simulink model "GammaandTorqueMover"  (R2022b)
settings: Solver=FixedStepAuto  StartTime=0.0  StopTime=10  FixedStep=0.01  RelTol=1e-3
undefined symbols (not defined in the file or in its folder): Kd, Ki, Kp
libraries: mpclib x6, slpidlib x6, simulink x1
(part 3 of 4)

== matlab function GammaandTorqueMover/PID/Subsystem/PINV/GAMMA ==
  data: input input; position input; output output; TAU input; BETA_K input; ALPHA_X input; ALPHA_Y input; ALPHA_Z input; ALPHA_M1 input; ALPHA_M2 input; BETA_M1 input; BETA_M2 input; ALPHA_RZ input; PI input
function output = computeGammaPinvBlock(input,position,TAU,BETA_K,ALPHA_X,ALPHA_Y,ALPHA_Z,ALPHA_M1,ALPHA_M2,BETA_M1,BETA_M2,ALPHA_RZ,PI)
    % Call the generated function to compute Gamma
    X_M = position(1);
    Y_M = position(2);
    Z_M = position(3);
    ALPHA_ROTATION_M = position(4);
    BETA_ROTATION_M = position(5);
    GAMMA_ROTATION_M = position(6);
    Gamma = computeFullGammawithTorqueR4(X_M,Y_M,Z_M,ALPHA_ROTATION_M,BETA_ROTATION_M,GAMMA_ROTATION_M,TAU,BETA_K,ALPHA_X,ALPHA_Y,ALPHA_Z,ALPHA_M1,ALPHA_M2,BETA_M1,BETA_M2,ALPHA_RZ,PI);
    Gamma_pinv = pinv(Gamma);
    
    % Multiply Gamma by the input
    output =Gamma_pinv * input ;
end

== matlab function GammaandTorqueMover/Open loop system/Subsystem/Gamma/GAMMA ==
  data: input input; position input; output output; TAU input; BETA_K input; ALPHA_X input; ALPHA_Y input; ALPHA_Z input; ALPHA_M1 input; ALPHA_M2 input; BETA_M1 input; BETA_M2 input; ALPHA_RZ input; PI input
function output = computeGammaBlock(input, position,TAU,BETA_K,ALPHA_X,ALPHA_Y,ALPHA_Z,ALPHA_M1,ALPHA_M2,BETA_M1,BETA_M2,ALPHA_RZ,PI)
% Call the generated function to compute Gamma
    X_M = position(1);
    Y_M = position(2);
    Z_M = position(3);
    ALPHA_ROTATION_M = position(4);
    BETA_ROTATION_M = position(5);
    GAMMA_ROTATION_M = position(6);
    Gamma = computeFullGammawithTorqueR4(X_M,Y_M,Z_M,ALPHA_ROTATION_M,BETA_ROTATION_M,GAMMA_ROTATION_M,TAU,BETA_K,ALPHA_X,ALPHA_Y,ALPHA_Z,ALPHA_M1,ALPHA_M2,BETA_M1,BETA_M2,ALPHA_RZ,PI);

    % Multiply Gamma by the input
    output = Gamma *input;
end

== matlab function GammaandTorqueMover/Open loop system/Subsystem/MATLAB Function ==
  data: xdot output; u input; y output; x input
function [xdot, y] = System_SS_Model(u, x)
    % Parameters
    m = 6.6;            % Mass (kg)
    g = 9.81;           % Gravitational acceleration (m/s^2)
    
    % Moment of Inertia
    Ixx = 0.059;        % Moment of inertia around x-axis
    Iyy = 0.059;        % Moment of inertia around y-axis
    Izz = 0.12;         % Moment of inertia around z-axis
    
    % State vector x = [Px, Vx, Py, Vy, Pz, Vz, α, ω_x, β, ω_y, γ, ω_z]
    % Input vector u = [Fx, Fy, Fz, Tx, Ty, Tz]
    
    % State-Space Matrix (continuous time)
    A = zeros(12, 12);
    % Position-velocity couplings
    A(1,2) = 1;  % Px dot = Vx
    A(3,4) = 1;  % Py dot = Vy
    A(5,6) = 1;  % Pz dot = Vz
    A(7,8) = 1;  % α dot = ω_x
    A(9,10) = 1; % β dot = ω_y
    A(11,12) = 1;% γ dot = ω_z
    
    % Input Matrix (continuous time)
    B = zeros(12, 6);
    % Force to acceleration conversion
    B(2,1) = 1/m;    % Fx -> ax
    B(4,2) = 1/m;    % Fy -> ay
    B(6,3) = 1/m;    % Fz -> az
    % Torque to angular acceleration conversion
    B(8,4) = 1/Ixx;  % Tx -> α_ddot
    B(10,5) = 1/Iyy; % Ty -> β_ddot
    B(12,6) = 1/Izz; % Tz -> γ_ddot
    
    % Gravitational effect (constant acceleration in z direction)
    gravity = zeros(12,1);
    gravity(6) = -g;  % Acceleration in z direction
    
    % State derivative (continuous time)
    xdot = A * x + B * u + gravity;
    
    % Output equation (we'll output all states)
    y = x;
end

== matlab function GammaandTorqueMover/Open loop system/Subsystem/PINV/GAMMA ==
  data: input input; position input; output output; TAU input; BETA_K input; ALPHA_X input; ALPHA_Y input; ALPHA_Z input; ALPHA_M1 input; ALPHA_M2 input; BETA_M1 input; BETA_M2 input; ALPHA_RZ input; PI input
function output = computeGammaPinvBlock(input,position,TAU,BETA_K,ALPHA_X,ALPHA_Y,ALPHA_Z,ALPHA_M1,ALPHA_M2,BETA_M1,BETA_M2,ALPHA_RZ,PI)
    % Call the generated function to compute Gamma
    X_M = position(1);
    Y_M = position(2);
    Z_M = position(3);
    ALPHA_ROTATION_M = position(4);
    BETA_ROTATION_M = position(5);
    GAMMA_ROTATION_M = position(6);
    Gamma = computeFullGammawithTorqueR4(X_M,Y_M,Z_M,ALPHA_ROTATION_M,BETA_ROTATION_M,GAMMA_ROTATION_M,TAU,BETA_K,ALPHA_X,ALPHA_Y,ALPHA_Z,ALPHA_M1,ALPHA_M2,BETA_M1,BETA_M2,ALPHA_RZ,PI);
    Gamma_pinv = pinv(Gamma);
    
    % Multiply Gamma by the input
    output =Gamma_pinv * input ;
end

== matlab function GammaandTorqueMover/Linear_MPC/MLPM Plant/Gamma/GAMMA ==
  data: input input; position input; output output; TAU input; BETA_K input; ALPHA_X input; ALPHA_Y input; ALPHA_Z input; ALPHA_M1 input; ALPHA_M2 input; BETA_M1 input; BETA_M2 input; ALPHA_RZ input; PI input
function output = computeGammaBlock(input, position,TAU,BETA_K,ALPHA_X,ALPHA_Y,ALPHA_Z,ALPHA_M1,ALPHA_M2,BETA_M1,BETA_M2,ALPHA_RZ,PI)
% Call the generated function to compute Gamma
    X_M = position(1);
    Y_M = position(2);
    Z_M = position(3);
    ALPHA_ROTATION_M = position(4);
    BETA_ROTATION_M = position(5);
    GAMMA_ROTATION_M = position(6);
    Gamma = computeFullGammawithTorqueR4(X_M,Y_M,Z_M,ALPHA_ROTATION_M,BETA_ROTATION_M,GAMMA_ROTATION_M,TAU,BETA_K,ALPHA_X,ALPHA_Y,ALPHA_Z,ALPHA_M1,ALPHA_M2,BETA_M1,BETA_M2,ALPHA_RZ,PI);

    % Multiply Gamma by the input
    output = Gamma *input;
end

== matlab function GammaandTorqueMover/Linear_MPC/MLPM Plant/MATLAB Function ==
  data: xdot output; u input; y output; x input
function [xdot, y] = System_SS_Model(u, x)
    % Parameters
    m = 6.6;            % Mass (kg)
    g = 9.81;           % Gravitational acceleration (m/s^2)
    
    % Moment of Inertia
    Ixx = 0.059;        % Moment of inertia around x-axis
    Iyy = 0.059;        % Moment of inertia around y-axis
    Izz = 0.12;         % Moment of inertia around z-axis
    
    % State vector x = [Px, Vx, Py, Vy, Pz, Vz, α, ω_x, β, ω_y, γ, ω_z]
    % Input vector u = [Fx, Fy, Fz, Tx, Ty, Tz]
    
    % State-Space Matrix (continuous time)
    A = zeros(12, 12);
    % Position-velocity couplings
    A(1,2) = 1;  % Px dot = Vx
    A(3,4) = 1;  % Py dot = Vy
    A(5,6) = 1;  % Pz dot = Vz
    A(7,8) = 1;  % α dot = ω_x
    A(9,10) = 1; % β dot = ω_y
    A(11,12) = 1;% γ dot = ω_z
    
    % Input Matrix (continuous time)
    B = zeros(12, 6);
    % Force to acceleration conversion
    B(2,1) = 1/m;    % Fx -> ax
    B(4,2) = 1/m;    % Fy -> ay
    B(6,3) = 1/m;    % Fz -> az
    % Torque to angular acceleration conversion
    B(8,4) = 1/Ixx;  % Tx -> α_ddot
    B(10,5) = 1/Iyy; % Ty -> β_ddot
    B(12,6) = 1/Izz; % Tz -> γ_ddot
    
    % Gravitational effect (constant acceleration in z direction)
    gravity = zeros(12,1);
    gravity(6) = -g;  % Acceleration in z direction
    
    % State derivative (continuous time)
    xdot = A * x + B * u + gravity;
    
    % Output equation: Only positions and orientations
    % Positions: Px (x(1)), Py (x(3)), Pz (x(5))
    % Orientations: α (x(7)), β (x(9)), γ (x(11))
    y = [ x(1); x(3); x(5); x(7); x(9); x(11) ];
end

== matlab function GammaandTorqueMover/Plant Verification/PINV/GAMMA ==
  data: input input; position input; output output; TAU input; BETA_K input; ALPHA_X input; ALPHA_Y input; ALPHA_Z input; ALPHA_M1 input; ALPHA_M2 input; BETA_M1 input; BETA_M2 input; ALPHA_RZ input; PI input
function output = computeGammaPinvBlock(input,position,TAU,BETA_K,ALPHA_X,ALPHA_Y,ALPHA_Z,ALPHA_M1,ALPHA_M2,BETA_M1,BETA_M2,ALPHA_RZ,PI)
    % Call the generated function to compute Gamma
    X_M = position(1);
    Y_M = position(2);
    Z_M = position(3);
    ALPHA_ROTATION_M = position(4);
    BETA_ROTATION_M = position(5);
    GAMMA_ROTATION_M = position(6);
    Gamma = computeFullGammawithTorqueR4(X_M,Y_M,Z_M,ALPHA_ROTATION_M,BETA_ROTATION_M,GAMMA_ROTATION_M,TAU,BETA_K,ALPHA_X,ALPHA_Y,ALPHA_Z,ALPHA_M1,ALPHA_M2,BETA_M1,BETA_M2,ALPHA_RZ,PI);
    Gamma_pinv = pinv(Gamma);
    
    % Multiply Gamma by the input
    output =Gamma_pinv * input ;
end

== matlab function GammaandTorqueMover/Linear_MPC/MLPM Plant/PINV/GAMMA ==
  data: input input; position input; output output; TAU input; BETA_K input; ALPHA_X input; ALPHA_Y input; ALPHA_Z input; ALPHA_M1 input; ALPHA_M2 input; BETA_M1 input; BETA_M2 input; ALPHA_RZ input; PI input
function output = computeGammaPinvBlock(input,position,TAU,BETA_K,ALPHA_X,ALPHA_Y,ALPHA_Z,ALPHA_M1,ALPHA_M2,BETA_M1,BETA_M2,ALPHA_RZ,PI)
    % Call the generated function to compute Gamma
    X_M = position(1);
    Y_M = position(2);
    Z_M = position(3);
    ALPHA_ROTATION_M = position(4);
    BETA_ROTATION_M = position(5);
    GAMMA_ROTATION_M = position(6);
    Gamma = computeFullGammawithTorqueR4(X_M,Y_M,Z_M,ALPHA_ROTATION_M,BETA_ROTATION_M,GAMMA_ROTATION_M,TAU,BETA_K,ALPHA_X,ALPHA_Y,ALPHA_Z,ALPHA_M1,ALPHA_M2,BETA_M1,BETA_M2,ALPHA_RZ,PI);
    Gamma_pinv = pinv(Gamma);
    
    % Multiply Gamma by the input
    output =Gamma_pinv * input ;
end

== matlab function GammaandTorqueMover/Mover Verification/MATLAB Function ==
  data: xdot output; u input; y output; x input
function [xdot, y] = System_SS_Model(u, x)
    % Parameters
    m = 6.6;            % Mass (kg)
    g = 9.81;           % Gravitational acceleration (m/s^2)
    
    % Moment of Inertia
    Ixx = 0.059;        % Moment of inertia around x-axis
    Iyy = 0.059;        % Moment of inertia around y-axis
    Izz = 0.12;         % Moment of inertia around z-axis
    
    % State vector x = [Px, Vx, Py, Vy, Pz, Vz, α, ω_x, β, ω_y, γ, ω_z]
    % Input vector u = [Fx, Fy, Fz, Tx, Ty, Tz]
    
    % State-Space Matrix (continuous time)
    A = zeros(12, 12);
    % Position-velocity couplings
    A(1,2) = 1;  % Px dot = Vx
    A(3,4) = 1;  % Py dot = Vy
    A(5,6) = 1;  % Pz dot = Vz
    A(7,8) = 1;  % α dot = ω_x
    A(9,10) = 1; % β dot = ω_y
    A(11,12) = 1;% γ dot = ω_z
    
    % Input Matrix (continuous time)
    B = zeros(12, 6);
    % Force to acceleration conversion
    B(2,1) = 1/m;    % Fx -> ax
    B(4,2) = 1/m;    % Fy -> ay
    B(6,3) = 1/m;    % Fz -> az
    % Torque to angular acceleration conversion
    B(8,4) = 1/Ixx;  % Tx -> α_ddot
    B(10,5) = 1/Iyy; % Ty -> β_ddot
    B(12,6) = 1/Izz; % Tz -> γ_ddot
    
    % Gravitational effect (constant acceleration in z direction)
    gravity = zeros(12,1);
    gravity(6) = -g;  % Acceleration in z direction
    
    % State derivative (continuous time)
    xdot = A * x + B * u + gravity;
    
    % Output equation (we'll output all states)
    y = x;
end

== matlab function GammaandTorqueMover/PID/MLPM Plant1/Gamma/GAMMA ==
  data: input input; position input; output output; TAU input; BETA_K input; ALPHA_X input; ALPHA_Y input; ALPHA_Z input; ALPHA_M1 input; ALPHA_M2 input; BETA_M1 input; BETA_M2 input; ALPHA_RZ input; PI input
function output = computeGammaBlock(input, position,TAU,BETA_K,ALPHA_X,ALPHA_Y,ALPHA_Z,ALPHA_M1,ALPHA_M2,BETA_M1,BETA_M2,ALPHA_RZ,PI)
% Call the generated function to compute Gamma
    X_M = position(1);
    Y_M = position(2);
    Z_M = position(3);
    ALPHA_ROTATION_M = position(4);
    BETA_ROTATION_M = position(5);
    GAMMA_ROTATION_M = position(6);
    Gamma = computeFullGammawithTorqueR4(X_M,Y_M,Z_M,ALPHA_ROTATION_M,BETA_ROTATION_M,GAMMA_ROTATION_M,TAU,BETA_K,ALPHA_X,ALPHA_Y,ALPHA_Z,ALPHA_M1,ALPHA_M2,BETA_M1,BETA_M2,ALPHA_RZ,PI);

    % Multiply Gamma by the input
    output = Gamma *input;
end

== matlab function GammaandTorqueMover/PID/MLPM Plant1/MATLAB Function ==
  data: xdot output; u input; y output; x input
function [xdot, y] = System_SS_Model(u,x)
    % Parameters
    m = 6.6;            % Mass (kg)
    dT = 0.01;           % Time step
    
    % Moment of Inertia (example values, should be calibrated to specific system)
    Ixx = 0.059;          % Moment of inertia around x-axis
    Iyy = 0.059;          % Moment of inertia around y-axis
    Izz = 0.12;         % Moment of inertia around z-axis
    
    % State vector x = [Px, Py, Pz, α, β, γ]
    % Input vector u = [Fx, Fy, Fz, Tx, Ty, Tz]
    
    % State-Space Matrix (positions and orientations only)
    A = [
        1, 0, 0, 0, 0, 0; % Px
        0, 1, 0, 0, 0, 0; % Py
        0, 0, 1, 0, 0, 0; % Pz
        0, 0, 0, 1, 0, 0; % α
        0, 0, 0, 0, 1, 0; % β
        0, 0, 0, 0, 0, 1; % γ
    ];
    
    % Input Matrix (positions and orientations only)
    B = [
        dT^2 / (2 * m), 0, 0, 0, 0, 0; % Px
        0, dT^2 / (2 * m), 0, 0, 0, 0; % Py
        0, 0, dT^2 / (2 * m), 0, 0, 0; % Pz
        0, 0, 0, dT^2 / (2 * Ixx), 0, 0; % α
        0, 0, 0, 0, dT^2 / (2 * Iyy), 0; % β
        0, 0, 0, 0, 0, dT^2 / (2 * Izz); % γ
    ];
    
    % Output Matrix (positions and orientations only)
    C = eye(6); % Direct mapping of states to outputs

    D = zeros(6, 6); % No direct feedthrough
    
    % State-Space equations
    xdot = A * x + B * u; % State derivative
    y = C * x + D *u;           % Output
end

== matlab function GammaandTorqueMover/PID/MLPM Plant1/PINV/GAMMA ==
  data: input input; position input; output output; TAU input; BETA_K input; ALPHA_X input; ALPHA_Y input; ALPHA_Z input; ALPHA_M1 input; ALPHA_M2 input; BETA_M1 input; BETA_M2 input; ALPHA_RZ input; PI input
function output = computeGammaPinvBlock(input,position,TAU,BETA_K,ALPHA_X,ALPHA_Y,ALPHA_Z,ALPHA_M1,ALPHA_M2,BETA_M1,BETA_M2,ALPHA_RZ,PI)
    % Call the generated function to compute Gamma
    X_M = position(1);
    Y_M = position(2);
    Z_M = position(3);
    ALPHA_ROTATION_M = position(4);
    BETA_ROTATION_M = position(5);
    GAMMA_ROTATION_M = position(6);
    Gamma = computeFullGammawithTorqueR4(X_M,Y_M,Z_M,ALPHA_ROTATION_M,BETA_ROTATION_M,GAMMA_ROTATION_M,TAU,BETA_K,ALPHA_X,ALPHA_Y,ALPHA_Z,ALPHA_M1,ALPHA_M2,BETA_M1,BETA_M2,ALPHA_RZ,PI);
    Gamma_pinv = pinv(Gamma);
    
    % Multiply Gamma by the input
    output =Gamma_pinv * input ;
end

== matlab function GammaandTorqueMover/PID2/Subsystem/Gamma/GAMMA ==
  data: input input; position input; output output; TAU input; BETA_K input; ALPHA_X input; ALPHA_Y input; ALPHA_Z input; ALPHA_M1 input; ALPHA_M2 input; BETA_M1 input; BETA_M2 input; ALPHA_RZ input; PI input
function output = computeGammaBlock(input, position,TAU,BETA_K,ALPHA_X,ALPHA_Y,ALPHA_Z,ALPHA_M1,ALPHA_M2,BETA_M1,BETA_M2,ALPHA_RZ,PI)
% Call the generated function to compute Gamma
    X_M = position(1);
    Y_M = position(2);
    Z_M = position(3);
    ALPHA_ROTATION_M = position(4);
    BETA_ROTATION_M = position(5);
    GAMMA_ROTATION_M = position(6);
    Gamma = computeFullGammawithTorqueR4(X_M,Y_M,Z_M,ALPHA_ROTATION_M,BETA_ROTATION_M,GAMMA_ROTATION_M,TAU,BETA_K,ALPHA_X,ALPHA_Y,ALPHA_Z,ALPHA_M1,ALPHA_M2,BETA_M1,BETA_M2,ALPHA_RZ,PI);

    % Multiply Gamma by the input
    output = Gamma *input;
end

== matlab function GammaandTorqueMover/PID2/Subsystem/MATLAB Function ==
  data: xdot output; u input; y output; x input
function [xdot, y] = System_SS_Model(u, x)
    % Parameters
    m = 6.6;            % Mass (kg)
    g = 9.81;           % Gravitational acceleration (m/s^2)
    
    % Moment of Inertia
    Ixx = 0.059;        % Moment of inertia around x-axis
    Iyy = 0.059;        % Moment of inertia around y-axis
    Izz = 0.12;         % Moment of inertia around z-axis
    
    % State vector x = [Px, Vx, Py, Vy, Pz, Vz, α, ω_x, β, ω_y, γ, ω_z]
    % Input vector u = [Fx, Fy, Fz, Tx, Ty, Tz]
    
    % State-Space Matrix (continuous time)
    A = zeros(12, 12);
    % Position-velocity couplings
    A(1,2) = 1;  % Px dot = Vx
    A(3,4) = 1;  % Py dot = Vy
    A(5,6) = 1;  % Pz dot = Vz
    A(7,8) = 1;  % α dot = ω_x
    A(9,10) = 1; % β dot = ω_y
    A(11,12) = 1;% γ dot = ω_z
    
    % Input Matrix (continuous time)
    B = zeros(12, 6);
    % Force to acceleration conversion
    B(2,1) = 1/m;    % Fx -> ax
    B(4,2) = 1/m;    % Fy -> ay
    B(6,3) = 1/m;    % Fz -> az
    % Torque to angular acceleration conversion
    B(8,4) = 1/Ixx;  % Tx -> α_ddot
    B(10,5) = 1/Iyy; % Ty -> β_ddot
    B(12,6) = 1/Izz; % Tz -> γ_ddot
    
    % Gravitational effect (constant acceleration in z direction)
    gravity = zeros(12,1);
    gravity(6) = -g;  % Acceleration in z direction
    
    % State derivative (continuous time)
    xdot = A * x + B * u + gravity;
    
    % Output equation (we'll output all states)
    y = x;
end

== matlab function GammaandTorqueMover/PID2/Subsystem/PINV/GAMMA ==
  data: input input; position input; output output; TAU input; BETA_K input; ALPHA_X input; ALPHA_Y input; ALPHA_Z input; ALPHA_M1 input; ALPHA_M2 input; BETA_M1 input; BETA_M2 input; ALPHA_RZ input; PI input
function output = computeGammaPinvBlock(input,position,TAU,BETA_K,ALPHA_X,ALPHA_Y,ALPHA_Z,ALPHA_M1,ALPHA_M2,BETA_M1,BETA_M2,ALPHA_RZ,PI)
    % Call the generated function to compute Gamma
    X_M = position(1);
    Y_M = position(2);
    Z_M = position(3);
    ALPHA_ROTATION_M = position(4);
    BETA_ROTATION_M = position(5);
    GAMMA_ROTATION_M = position(6);
    Gamma = computeFullGammawithTorqueR4(X_M,Y_M,Z_M,ALPHA_ROTATION_M,BETA_ROTATION_M,GAMMA_ROTATION_M,TAU,BETA_K,ALPHA_X,ALPHA_Y,ALPHA_Z,ALPHA_M1,ALPHA_M2,BETA_M1,BETA_M2,ALPHA_RZ,PI);
    Gamma_pinv = pinv(Gamma);
    
    % Multiply Gamma by the input
    output =Gamma_pinv * input ;
end

== matlab function GammaandTorqueMover/Linear MPC/MLPM Plant1/Gamma/GAMMA ==
  data: input input; position input; output output; TAU input; BETA_K input; ALPHA_X input; ALPHA_Y input; ALPHA_Z input; ALPHA_M1 input; ALPHA_M2 input; BETA_M1 input; BETA_M2 input; ALPHA_RZ input; PI input
function output = computeGammaBlock(input, position,TAU,BETA_K,ALPHA_X,ALPHA_Y,ALPHA_Z,ALPHA_M1,ALPHA_M2,BETA_M1,BETA_M2,ALPHA_RZ,PI)
% Call the generated function to compute Gamma
    X_M = position(1);
    Y_M = position(2);
    Z_M = position(3);
    ALPHA_ROTATION_M = position(4);
    BETA_ROTATION_M = position(5);
    GAMMA_ROTATION_M = position(6);
    Gamma = computeFullGammawithTorqueR4(X_M,Y_M,Z_M,ALPHA_ROTATION_M,BETA_ROTATION_M,GAMMA_ROTATION_M,TAU,BETA_K,ALPHA_X,ALPHA_Y,ALPHA_Z,ALPHA_M1,ALPHA_M2,BETA_M1,BETA_M2,ALPHA_RZ,PI);

    % Multiply Gamma by the input
    output = Gamma *input;
end

== matlab function GammaandTorqueMover/Linear MPC/MLPM Plant1/MATLAB Function ==
  data: xdot output; u input; y output; x input
function [xdot, y] = System_SS_Model(u,x)
    % Parameters
    m = 6.6;            % Mass (kg)
    dT = 0.01;           % Time step
    
    % Moment of Inertia (example values, should be calibrated to specific system)
    Ixx = 0.059;          % Moment of inertia around x-axis
    Iyy = 0.059;          % Moment of inertia around y-axis
    Izz = 0.12;         % Moment of inertia around z-axis
    
    % State vector x = [Px, Py, Pz, α, β, γ]
    % Input vector u = [Fx, Fy, Fz, Tx, Ty, Tz]
    
    % State-Space Matrix (positions and orientations only)
    A = [
        1, 0, 0, 0, 0, 0; % Px
        0, 1, 0, 0, 0, 0; % Py
        0, 0, 1, 0, 0, 0; % Pz
        0, 0, 0, 1, 0, 0; % α
        0, 0, 0, 0, 1, 0; % β
        0, 0, 0, 0, 0, 1; % γ
    ];
    
    % Input Matrix (positions and orientations only)
    B = [
        dT^2 / (2 * m), 0, 0, 0, 0, 0; % Px
        0, dT^2 / (2 * m), 0, 0, 0, 0; % Py
        0, 0, dT^2 / (2 * m), 0, 0, 0; % Pz
        0, 0, 0, dT^2 / (2 * Ixx), 0, 0; % α
        0, 0, 0, 0, dT^2 / (2 * Iyy), 0; % β
        0, 0, 0, 0, 0, dT^2 / (2 * Izz); % γ
    ];
    
    % Output Matrix (positions and orientations only)
    C = eye(6); % Direct mapping of states to outputs

    D = zeros(6, 6); % No direct feedthrough
    
    % State-Space equations
    xdot = A * x + B * u; % State derivative
    y = C * x + D *u;           % Output
end

== matlab function GammaandTorqueMover/Linear MPC/MLPM Plant1/PINV/GAMMA ==
  data: input input; position input; output output; TAU input; BETA_K input; ALPHA_X input; ALPHA_Y input; ALPHA_Z input; ALPHA_M1 input; ALPHA_M2 input; BETA_M1 input; BETA_M2 input; ALPHA_RZ input; PI input
function output = computeGammaPinvBlock(input,position,TAU,BETA_K,ALPHA_X,ALPHA_Y,ALPHA_Z,ALPHA_M1,ALPHA_M2,BETA_M1,BETA_M2,ALPHA_RZ,PI)
    % Call the generated function to compute Gamma
    X_M = position(1);
    Y_M = position(2);
    Z_M = position(3);
    ALPHA_ROTATION_M = position(4);
    BETA_ROTATION_M = position(5);
    GAMMA_ROTATION_M = position(6);
    Gamma = computeFullGammawithTorqueR4(X_M,Y_M,Z_M,ALPHA_ROTATION_M,BETA_ROTATION_M,GAMMA_ROTATION_M,TAU,BETA_K,ALPHA_X,ALPHA_Y,ALPHA_Z,ALPHA_M1,ALPHA_M2,BETA_M1,BETA_M2,ALPHA_RZ,PI);
    Gamma_pinv = pinv(Gamma);
    
    % Multiply Gamma by the input
    output =Gamma_pinv * input ;
end

== matlab function GammaandTorqueMover/Linear MPC/Subsystem/Gamma/GAMMA ==
  data: input input; position input; output output; TAU input; BETA_K input; ALPHA_X input; ALPHA_Y input; ALPHA_Z input; ALPHA_M1 input; ALPHA_M2 input; BETA_M1 input; BETA_M2 input; ALPHA_RZ input; PI input
function output = computeGammaBlock(input, position,TAU,BETA_K,ALPHA_X,ALPHA_Y,ALPHA_Z,ALPHA_M1,ALPHA_M2,BETA_M1,BETA_M2,ALPHA_RZ,PI)
% Call the generated function to compute Gamma
    X_M = position(1);
    Y_M = position(2);
    Z_M = position(3);
    ALPHA_ROTATION_M = position(4);
    BETA_ROTATION_M = position(5);
    GAMMA_ROTATION_M = position(6);
    Gamma = computeFullGammawithTorqueR4(X_M,Y_M,Z_M,ALPHA_ROTATION_M,BETA_ROTATION_M,GAMMA_ROTATION_M,TAU,BETA_K,ALPHA_X,ALPHA_Y,ALPHA_Z,ALPHA_M1,ALPHA_M2,BETA_M1,BETA_M2,ALPHA_RZ,PI);

    % Multiply Gamma by the input
    output = Gamma *input;
end

== matlab function GammaandTorqueMover/Plant Verification/MATLAB Function ==
  data: xdot output; u input; y output; x input
function [xdot, y] = System_SS_Model(u, x)
    % Parameters
    m = 6.6;            % Mass (kg)
    g = 9.81;           % Gravitational acceleration (m/s^2)
    
    % Moment of Inertia
    Ixx = 0.059;        % Moment of inertia around x-axis
    Iyy = 0.059;        % Moment of inertia around y-axis
    Izz = 0.12;         % Moment of inertia around z-axis
    
    % State vector x = [Px, Vx, Py, Vy, Pz, Vz, α, ω_x, β, ω_y, γ, ω_z]
    % Input vector u = [Fx, Fy, Fz, Tx, Ty, Tz]
    
    % State-Space Matrix (continuous time)
    A = zeros(12, 12);
    % Position-velocity couplings
    A(1,2) = 1;  % Px dot = Vx
    A(3,4) = 1;  % Py dot = Vy
    A(5,6) = 1;  % Pz dot = Vz
    A(7,8) = 1;  % α dot = ω_x
    A(9,10) = 1; % β dot = ω_y
    A(11,12) = 1;% γ dot = ω_z
    
    % Input Matrix (continuous time)
    B = zeros(12, 6);
    % Force to acceleration conversion
    B(2,1) = 1/m;    % Fx -> ax
    B(4,2) = 1/m;    % Fy -> ay
    B(6,3) = 1/m;    % Fz -> az
    % Torque to angular acceleration conversion
    B(8,4) = 1/Ixx;  % Tx -> α_ddot
    B(10,5) = 1/Iyy; % Ty -> β_ddot
    B(12,6) = 1/Izz; % Tz -> γ_ddot
    
    % Gravitational effect (constant acceleration in z direction)
    gravity = zeros(12,1);
    gravity(6) = -g;  % Acceleration in z direction
    
    % State derivative (continuous time)
    xdot = A * x + B * u + gravity;
    
    % Output equation (we'll output all states)
    y = x;
end

== matlab function GammaandTorqueMover/Linear MPC/Subsystem/MATLAB Function ==
  data: xdot output; u input; y output; x input
function [xdot, y] = System_SS_Model(u, x)
    % Parameters
    m = 6.6;            % Mass (kg)
    g = 9.81;           % Gravitational acceleration (m/s^2)
    
    % Moment of Inertia
    Ixx = 0.059;        % Moment of inertia around x-axis
    Iyy = 0.059;        % Moment of inertia around y-axis
    Izz = 0.12;         % Moment of inertia around z-axis
    
    % State vector x = [Px, Vx, Py, Vy, Pz, Vz, α, ω_x, β, ω_y, γ, ω_z]
    % Input vector u = [Fx, Fy, Fz, Tx, Ty, Tz]
    
    % State-Space Matrix (continuous time)
    A = zeros(12, 12);
    % Position-velocity couplings
    A(1,2) = 1;  % Px dot = Vx
    A(3,4) = 1;  % Py dot = Vy
    A(5,6) = 1;  % Pz dot = Vz
    A(7,8) = 1;  % α dot = ω_x
    A(9,10) = 1; % β dot = ω_y
    A(11,12) = 1;% γ dot = ω_z
    
    % Input Matrix (continuous time)
    B = zeros(12, 6);
    % Force to acceleration conversion
    B(2,1) = 1/m;    % Fx -> ax
    B(4,2) = 1/m;    % Fy -> ay
    B(6,3) = 1/m;    % Fz -> az
    % Torque to angular acceleration conversion
    B(8,4) = 1/Ixx;  % Tx -> α_ddot
    B(10,5) = 1/Iyy; % Ty -> β_ddot
    B(12,6) = 1/Izz; % Tz -> γ_ddot
    
    % Gravitational effect (constant acceleration in z direction)
    gravity = zeros(12,1);
    gravity(6) = -g;  % Acceleration in z direction
    
    % State derivative (continuous time)
    xdot = A * x + B * u + gravity;
    
    % Output equation: Only positions and orientations
    % Positions: Px (x(1)), Py (x(3)), Pz (x(5))
    % Orientations: α (x(7)), β (x(9)), γ (x(11))
    y = [ x(1); x(3); x(5); x(7); x(9); x(11) ];
end

== matlab function GammaandTorqueMover/Linear MPC/Subsystem/PINV/GAMMA ==
  data: input input; position input; output output; TAU input; BETA_K input; ALPHA_X input; ALPHA_Y input; ALPHA_Z input; ALPHA_M1 input; ALPHA_M2 input; BETA_M1 input; BETA_M2 input; ALPHA_RZ input; PI input
function output = computeGammaPinvBlock(input,position,TAU,BETA_K,ALPHA_X,ALPHA_Y,ALPHA_Z,ALPHA_M1,ALPHA_M2,BETA_M1,BETA_M2,ALPHA_RZ,PI)
    % Call the generated function to compute Gamma
    X_M = position(1);
    Y_M = position(2);
    Z_M = position(3);
    ALPHA_ROTATION_M = position(4);
    BETA_ROTATION_M = position(5);
    GAMMA_ROTATION_M = position(6);
    Gamma = computeFullGammawithTorqueR4(X_M,Y_M,Z_M,ALPHA_ROTATION_M,BETA_ROTATION_M,GAMMA_ROTATION_M,TAU,BETA_K,ALPHA_X,ALPHA_Y,ALPHA_Z,ALPHA_M1,ALPHA_M2,BETA_M1,BETA_M2,ALPHA_RZ,PI);
    Gamma_pinv = pinv(Gamma);
    
    % Multiply Gamma by the input
    output =Gamma_pinv * input ;
end

== matlab function GammaandTorqueMover/PID1/MLPM Plant1/Gamma/GAMMA ==
  data: input input; position input; output output; TAU input; BETA_K input; ALPHA_X input; ALPHA_Y input; ALPHA_Z input; ALPHA_M1 input; ALPHA_M2 input; BETA_M1 input; BETA_M2 input; ALPHA_RZ input; PI input
function output = computeGammaBlock(input, position,TAU,BETA_K,ALPHA_X,ALPHA_Y,ALPHA_Z,ALPHA_M1,ALPHA_M2,BETA_M1,BETA_M2,ALPHA_RZ,PI)
% Call the generated function to compute Gamma
    X_M = position(1);
    Y_M = position(2);
    Z_M = position(3);
    ALPHA_ROTATION_M = position(4);
    BETA_ROTATION_M = position(5);
    GAMMA_ROTATION_M = position(6);
    Gamma = computeFullGammawithTorqueR4(X_M,Y_M,Z_M,ALPHA_ROTATION_M,BETA_ROTATION_M,GAMMA_ROTATION_M,TAU,BETA_K,ALPHA_X,ALPHA_Y,ALPHA_Z,ALPHA_M1,ALPHA_M2,BETA_M1,BETA_M2,ALPHA_RZ,PI);

    % Multiply Gamma by the input
    output = Gamma *input;
end

== matlab function GammaandTorqueMover/PID1/MLPM Plant1/MATLAB Function ==
  data: xdot output; u input; y output; x input
function [xdot, y] = System_SS_Model(u,x)
    % Parameters
    m = 6.6;            % Mass (kg)
    dT = 0.01;           % Time step
    
    % Moment of Inertia (example values, should be calibrated to specific system)
    Ixx = 0.059;          % Moment of inertia around x-axis
    Iyy = 0.059;          % Moment of inertia around y-axis
    Izz = 0.12;         % Moment of inertia around z-axis
    
    % State vector x = [Px, Py, Pz, α, β, γ]
    % Input vector u = [Fx, Fy, Fz, Tx, Ty, Tz]
    
    % State-Space Matrix (positions and orientations only)
    A = [
        1, 0, 0, 0, 0, 0; % Px
        0, 1, 0, 0, 0, 0; % Py
        0, 0, 1, 0, 0, 0; % Pz
        0, 0, 0, 1, 0, 0; % α
        0, 0, 0, 0, 1, 0; % β
        0, 0, 0, 0, 0, 1; % γ
    ];
    
    % Input Matrix (positions and orientations only)
    B = [
        dT^2 / (2 * m), 0, 0, 0, 0, 0; % Px
        0, dT^2 / (2 * m), 0, 0, 0, 0; % Py
        0, 0, dT^2 / (2 * m), 0, 0, 0; % Pz
        0, 0, 0, dT^2 / (2 * Ixx), 0, 0; % α
        0, 0, 0, 0, dT^2 / (2 * Iyy), 0; % β
        0, 0, 0, 0, 0, dT^2 / (2 * Izz); % γ
    ];
    
    % Output Matrix (positions and orientations only)
    C = eye(6); % Direct mapping of states to outputs

    D = zeros(6, 6); % No direct feedthrough
    
    % State-Space equations
    xdot = A * x + B * u; % State derivative
    y = C * x + D *u;           % Output
end

== matlab function GammaandTorqueMover/PID1/MLPM Plant1/PINV/GAMMA ==
  data: input input; position input; output output; TAU input; BETA_K input; ALPHA_X input; ALPHA_Y input; ALPHA_Z input; ALPHA_M1 input; ALPHA_M2 input; BETA_M1 input; BETA_M2 input; ALPHA_RZ input; PI input
function output = computeGammaPinvBlock(input,position,TAU,BETA_K,ALPHA_X,ALPHA_Y,ALPHA_Z,ALPHA_M1,ALPHA_M2,BETA_M1,BETA_M2,ALPHA_RZ,PI)
    % Call the generated function to compute Gamma
    X_M = position(1);
    Y_M = position(2);
    Z_M = position(3);
    ALPHA_ROTATION_M = position(4);
    BETA_ROTATION_M = position(5);
    GAMMA_ROTATION_M = position(6);
    Gamma = computeFullGammawithTorqueR4(X_M,Y_M,Z_M,ALPHA_ROTATION_M,BETA_ROTATION_M,GAMMA_ROTATION_M,TAU,BETA_K,ALPHA_X,ALPHA_Y,ALPHA_Z,ALPHA_M1,ALPHA_M2,BETA_M1,BETA_M2,ALPHA_RZ,PI);
    Gamma_pinv = pinv(Gamma);
    
    % Multiply Gamma by the input
    output =Gamma_pinv * input ;
end

== matlab function GammaandTorqueMover/PID1/Subsystem/Gamma/GAMMA ==
  data: input input; position input; output output; TAU input; BETA_K input; ALPHA_X input; ALPHA_Y input; ALPHA_Z input; ALPHA_M1 input; ALPHA_M2 input; BETA_M1 input; BETA_M2 input; ALPHA_RZ input; PI input
function output = computeGammaBlock(input, position,TAU,BETA_K,ALPHA_X,ALPHA_Y,ALPHA_Z,ALPHA_M1,ALPHA_M2,BETA_M1,BETA_M2,ALPHA_RZ,PI)
% Call the generated function to compute Gamma
    X_M = position(1);
    Y_M = position(2);
    Z_M = position(3);
    ALPHA_ROTATION_M = position(4);
    BETA_ROTATION_M = position(5);
    GAMMA_ROTATION_M = position(6);
    Gamma = computeFullGammawithTorqueR4(X_M,Y_M,Z_M,ALPHA_ROTATION_M,BETA_ROTATION_M,GAMMA_ROTATION_M,TAU,BETA_K,ALPHA_X,ALPHA_Y,ALPHA_Z,ALPHA_M1,ALPHA_M2,BETA_M1,BETA_M2,ALPHA_RZ,PI);

    % Multiply Gamma by the input
    output = Gamma *input;
end

== matlab function GammaandTorqueMover/Linear MPC old/Gamma/GAMMA ==
  data: input input; X_M input; output output; Y_M input; Z_M input; TAU input; BETA_K input; ALPHA_X input; ALPHA_Y input; ALPHA_Z input; ALPHA_M1 input; ALPHA_M2 input; BETA_M1 input; BETA_M2 input; ALPHA_RZ input; PI input
function output = computeGammaBlock(input, X_M,Y_M,Z_M,TAU,BETA_K,ALPHA_X,ALPHA_Y,ALPHA_Z,ALPHA_M1,ALPHA_M2,BETA_M1,BETA_M2,ALPHA_RZ,PI)
    % Call the generated function to compute Gamma
    Gamma = computeFullGammawithTorque3(X_M,Y_M,Z_M,TAU,BETA_K,ALPHA_X,ALPHA_Y,ALPHA_Z,ALPHA_M1,ALPHA_M2,BETA_M1,BETA_M2,ALPHA_RZ,PI);
    
    % Multiply Gamma by the input
    output = Gamma * input;
end

== matlab function GammaandTorqueMover/PID1/Subsystem/MATLAB Function ==
  data: xdot output; u input; y output; x input
function [xdot, y] = System_SS_Model(u, x)
    % Parameters
    m = 6.6;            % Mass (kg)
    g = 9.81;           % Gravitational acceleration (m/s^2)
    
    % Moment of Inertia
    Ixx = 0.059;        % Moment of inertia around x-axis
    Iyy = 0.059;        % Moment of inertia around y-axis
    Izz = 0.12;         % Moment of inertia around z-axis
    
    % State vector x = [Px, Vx, Py, Vy, Pz, Vz, α, ω_x, β, ω_y, γ, ω_z]
    % Input vector u = [Fx, Fy, Fz, Tx, Ty, Tz]
    
    % State-Space Matrix (continuous time)
    A = zeros(12, 12);
    % Position-velocity couplings
    A(1,2) = 1;  % Px dot = Vx
    A(3,4) = 1;  % Py dot = Vy
    A(5,6) = 1;  % Pz dot = Vz
    A(7,8) = 1;  % α dot = ω_x
    A(9,10) = 1; % β dot = ω_y
    A(11,12) = 1;% γ dot = ω_z
    
    % Input Matrix (continuous time)
    B = zeros(12, 6);
    % Force to acceleration conversion
    B(2,1) = 1/m;    % Fx -> ax
    B(4,2) = 1/m;    % Fy -> ay
    B(6,3) = 1/m;    % Fz -> az
    % Torque to angular acceleration conversion
    B(8,4) = 1/Ixx;  % Tx -> α_ddot
    B(10,5) = 1/Iyy; % Ty -> β_ddot
    B(12,6) = 1/Izz; % Tz -> γ_ddot
    
    % Gravitational effect (constant acceleration in z direction)
    gravity = zeros(12,1);
    gravity(6) = -g;  % Acceleration in z direction
    
    % State derivative (continuous time)
    xdot = A * x + B * u + gravity;
    
    % Output equation: Only positions and orientations
    % Positions: Px (x(1)), Py (x(3)), Pz (x(5))
    % Orientations: α (x(7)), β (x(9)), γ (x(11))
    y = [ x(1); x(3); x(5); x(7); x(9); x(11) ];
end

== matlab function GammaandTorqueMover/PID1/Subsystem/PINV/GAMMA ==
  data: input input; position input; output output; TAU input; BETA_K input; ALPHA_X input; ALPHA_Y input; ALPHA_Z input; ALPHA_M1 input; ALPHA_M2 input; BETA_M1 input; BETA_M2 input; ALPHA_RZ input; PI input
function output = computeGammaPinvBlock(input,position,TAU,BETA_K,ALPHA_X,ALPHA_Y,ALPHA_Z,ALPHA_M1,ALPHA_M2,BETA_M1,BETA_M2,ALPHA_RZ,PI)
    % Call the generated function to compute Gamma
    X_M = position(1);
    Y_M = position(2);
    Z_M = position(3);
    ALPHA_ROTATION_M = position(4);
    BETA_ROTATION_M = position(5);
    GAMMA_ROTATION_M = position(6);
    Gamma = computeFullGammawithTorqueR4(X_M,Y_M,Z_M,ALPHA_ROTATION_M,BETA_ROTATION_M,GAMMA_ROTATION_M,TAU,BETA_K,ALPHA_X,ALPHA_Y,ALPHA_Z,ALPHA_M1,ALPHA_M2,BETA_M1,BETA_M2,ALPHA_RZ,PI);
    Gamma_pinv = pinv(Gamma);
    
    % Multiply Gamma by the input
    output =Gamma_pinv * input ;
end

== matlab function GammaandTorqueMover/Tube MPC/MLPM Plant1/Gamma/GAMMA ==
  data: input input; position input; output output; TAU input; BETA_K input; ALPHA_X input; ALPHA_Y input; ALPHA_Z input; ALPHA_M1 input; ALPHA_M2 input; BETA_M1 input; BETA_M2 input; ALPHA_RZ input; PI input
function output = computeGammaBlock(input, position,TAU,BETA_K,ALPHA_X,ALPHA_Y,ALPHA_Z,ALPHA_M1,ALPHA_M2,BETA_M1,BETA_M2,ALPHA_RZ,PI)
% Call the generated function to compute Gamma
    X_M = position(1);
    Y_M = position(2);
    Z_M = position(3);
    ALPHA_ROTATION_M = position(4);
    BETA_ROTATION_M = position(5);
    GAMMA_ROTATION_M = position(6);
    Gamma = computeFullGammawithTorqueR4(X_M,Y_M,Z_M,ALPHA_ROTATION_M,BETA_ROTATION_M,GAMMA_ROTATION_M,TAU,BETA_K,ALPHA_X,ALPHA_Y,ALPHA_Z,ALPHA_M1,ALPHA_M2,BETA_M1,BETA_M2,ALPHA_RZ,PI);

    % Multiply Gamma by the input
    output = Gamma *input;
end

== matlab function GammaandTorqueMover/Tube MPC/MLPM Plant1/MATLAB Function ==
  data: xdot output; u input; y output; x input
function [xdot, y] = System_SS_Model(u,x)
    % Parameters
    m = 6.6;            % Mass (kg)
    dT = 0.01;           % Time step
    
    % Moment of Inertia (example values, should be calibrated to specific system)
    Ixx = 0.059;          % Moment of inertia around x-axis
    Iyy = 0.059;          % Moment of inertia around y-axis
    Izz = 0.12;         % Moment of inertia around z-axis
    
    % State vector x = [Px, Py, Pz, α, β, γ]
    % Input vector u = [Fx, Fy, Fz, Tx, Ty, Tz]
    
    % State-Space Matrix (positions and orientations only)
    A = [
        1, 0, 0, 0, 0, 0; % Px
        0, 1, 0, 0, 0, 0; % Py
        0, 0, 1, 0, 0, 0; % Pz
        0, 0, 0, 1, 0, 0; % α
        0, 0, 0, 0, 1, 0; % β
        0, 0, 0, 0, 0, 1; % γ
    ];
    
    % Input Matrix (positions and orientations only)
    B = [
        dT^2 / (2 * m), 0, 0, 0, 0, 0; % Px
        0, dT^2 / (2 * m), 0, 0, 0, 0; % Py
        0, 0, dT^2 / (2 * m), 0, 0, 0; % Pz
        0, 0, 0, dT^2 / (2 * Ixx), 0, 0; % α
        0, 0, 0, 0, dT^2 / (2 * Iyy), 0; % β
        0, 0, 0, 0, 0, dT^2 / (2 * Izz); % γ
    ];
    
    % Output Matrix (positions and orientations only)
    C = eye(6); % Direct mapping of states to outputs

    D = zeros(6, 6); % No direct feedthrough
    
    % State-Space equations
    xdot = A * x + B * u; % State derivative
    y = C * x + D *u;           % Output
end

== matlab function GammaandTorqueMover/Tube MPC/MLPM Plant1/PINV/GAMMA ==
  data: input input; position input; output output; TAU input; BETA_K input; ALPHA_X input; ALPHA_Y input; ALPHA_Z input; ALPHA_M1 input; ALPHA_M2 input; BETA_M1 input; BETA_M2 input; ALPHA_RZ input; PI input
function output = computeGammaPinvBlock(input,position,TAU,BETA_K,ALPHA_X,ALPHA_Y,ALPHA_Z,ALPHA_M1,ALPHA_M2,BETA_M1,BETA_M2,ALPHA_RZ,PI)
    % Call the generated function to compute Gamma
    X_M = position(1);
    Y_M = position(2);
    Z_M = position(3);
    ALPHA_ROTATION_M = position(4);
    BETA_ROTATION_M = position(5);
    GAMMA_ROTATION_M = position(6);
    Gamma = computeFullGammawithTorqueR4(X_M,Y_M,Z_M,ALPHA_ROTATION_M,BETA_ROTATION_M,GAMMA_ROTATION_M,TAU,BETA_K,ALPHA_X,ALPHA_Y,ALPHA_Z,ALPHA_M1,ALPHA_M2,BETA_M1,BETA_M2,ALPHA_RZ,PI);
    Gamma_pinv = pinv(Gamma);
    
    % Multiply Gamma by the input
    output =Gamma_pinv * input ;
end

== matlab function GammaandTorqueMover/Tube MPC/Subsystem/Gamma/GAMMA ==
  data: input input; position input; output output; TAU input; BETA_K input; ALPHA_X input; ALPHA_Y input; ALPHA_Z input; ALPHA_M1 input; ALPHA_M2 input; BETA_M1 input; BETA_M2 input; ALPHA_RZ input; PI input
function output = computeGammaBlock(input, position,TAU,BETA_K,ALPHA_X,ALPHA_Y,ALPHA_Z,ALPHA_M1,ALPHA_M2,BETA_M1,BETA_M2,ALPHA_RZ,PI)
% Call the generated function to compute Gamma
    X_M = position(1);
    Y_M = position(2);
    Z_M = position(3);
    ALPHA_ROTATION_M = position(4);
    BETA_ROTATION_M = position(5);
    GAMMA_ROTATION_M = position(6);
    Gamma = computeFullGammawithTorqueR4(X_M,Y_M,Z_M,ALPHA_ROTATION_M,BETA_ROTATION_M,GAMMA_ROTATION_M,TAU,BETA_K,ALPHA_X,ALPHA_Y,ALPHA_Z,ALPHA_M1,ALPHA_M2,BETA_M1,BETA_M2,ALPHA_RZ,PI);

    % Multiply Gamma by the input
    output = Gamma *input;
end

== matlab function GammaandTorqueMover/Tube MPC/Subsystem/MATLAB Function ==
  data: xdot output; u input; y output; x input
function [xdot, y] = System_SS_Model(u, x)
    % Parameters
    m = 6.6;            % Mass (kg)
    g = 9.81;           % Gravitational acceleration (m/s^2)
    
    % Moment of Inertia
    Ixx = 0.059;        % Moment of inertia around x-axis
    Iyy = 0.059;        % Moment of inertia around y-axis
    Izz = 0.12;         % Moment of inertia around z-axis
    
    % State vector x = [Px, Vx, Py, Vy, Pz, Vz, α, ω_x, β, ω_y, γ, ω_z]
    % Input vector u = [Fx, Fy, Fz, Tx, Ty, Tz]
    
    % State-Space Matrix (continuous time)
    A = zeros(12, 12);
    % Position-velocity couplings
    A(1,2) = 1;  % Px dot = Vx
    A(3,4) = 1;  % Py dot = Vy
    A(5,6) = 1;  % Pz dot = Vz
    A(7,8) = 1;  % α dot = ω_x
    A(9,10) = 1; % β dot = ω_y
    A(11,12) = 1;% γ dot = ω_z
    
    % Input Matrix (continuous time)
    B = zeros(12, 6);
    % Force to acceleration conversion
    B(2,1) = 1/m;    % Fx -> ax
    B(4,2) = 1/m;    % Fy -> ay
    B(6,3) = 1/m;    % Fz -> az
    % Torque to angular acceleration conversion
    B(8,4) = 1/Ixx;  % Tx -> α_ddot
    B(10,5) = 1/Iyy; % Ty -> β_ddot
    B(12,6) = 1/Izz; % Tz -> γ_ddot
    
    % Gravitational effect (constant acceleration in z direction)
    gravity = zeros(12,1);
    gravity(6) = -g;  % Acceleration in z direction
    
    % State derivative (continuous time)
    xdot = A * x + B * u + gravity;
    
    % Output equation: Only positions and orientations
    % Positions: Px (x(1)), Py (x(3)), Pz (x(5))
    % Orientations: α (x(7)), β (x(9)), γ (x(11))
    y = [ x(1); x(3); x(5); x(7); x(9); x(11) ];
end

== matlab function GammaandTorqueMover/Tube MPC/Subsystem/PINV/GAMMA ==
  data: input input; position input; output output; TAU input; BETA_K input; ALPHA_X input; ALPHA_Y input; ALPHA_Z input; ALPHA_M1 input; ALPHA_M2 input; BETA_M1 input; BETA_M2 input; ALPHA_RZ input; PI input
function output = computeGammaPinvBlock(input,position,TAU,BETA_K,ALPHA_X,ALPHA_Y,ALPHA_Z,ALPHA_M1,ALPHA_M2,BETA_M1,BETA_M2,ALPHA_RZ,PI)
    % Call the generated function to compute Gamma
    X_M = position(1);
    Y_M = position(2);
    Z_M = position(3);
    ALPHA_ROTATION_M = position(4);
    BETA_ROTATION_M = position(5);
    GAMMA_ROTATION_M = position(6);
    Gamma = computeFullGammawithTorqueR4(X_M,Y_M,Z_M,ALPHA_ROTATION_M,BETA_ROTATION_M,GAMMA_ROTATION_M,TAU,BETA_K,ALPHA_X,ALPHA_Y,ALPHA_Z,ALPHA_M1,ALPHA_M2,BETA_M1,BETA_M2,ALPHA_RZ,PI);
    Gamma_pinv = pinv(Gamma);
    
    % Multiply Gamma by the input
    output =Gamma_pinv * input ;
end

== matlab function GammaandTorqueMover/Disturbance added/Linear MPC plus D/MLPM Plant1/Gamma/GAMMA ==
  data: input input; position input; output output; TAU input; BETA_K input; ALPHA_X input; ALPHA_Y input; ALPHA_Z input; ALPHA_M1 input; ALPHA_M2 input; BETA_M1 input; BETA_M2 input; ALPHA_RZ input; PI input
function output = computeGammaBlock(input, position,TAU,BETA_K,ALPHA_X,ALPHA_Y,ALPHA_Z,ALPHA_M1,ALPHA_M2,BETA_M1,BETA_M2,ALPHA_RZ,PI)
% Call the generated function to compute Gamma
    X_M = position(1);
    Y_M = position(2);
    Z_M = position(3);
    ALPHA_ROTATION_M = position(4);
    BETA_ROTATION_M = position(5);
    GAMMA_ROTATION_M = position(6);
    Gamma = computeFullGammawithTorqueR4(X_M,Y_M,Z_M,ALPHA_ROTATION_M,BETA_ROTATION_M,GAMMA_ROTATION_M,TAU,BETA_K,ALPHA_X,ALPHA_Y,ALPHA_Z,ALPHA_M1,ALPHA_M2,BETA_M1,BETA_M2,ALPHA_RZ,PI);

    % Multiply Gamma by the input
    output = Gamma *input;
end

== matlab function GammaandTorqueMover/Disturbance added/Linear MPC plus D/MLPM Plant1/MATLAB Function ==
  data: xdot output; u input; y output; x input
function [xdot, y] = System_SS_Model(u,x)
    % Parameters
    m = 6.6;            % Mass (kg)
    dT = 0.01;           % Time step
    
    % Moment of Inertia (example values, should be calibrated to specific system)
    Ixx = 0.059;          % Moment of inertia around x-axis
    Iyy = 0.059;          % Moment of inertia around y-axis
    Izz = 0.12;         % Moment of inertia around z-axis
    
    % State vector x = [Px, Py, Pz, α, β, γ]
    % Input vector u = [Fx, Fy, Fz, Tx, Ty, Tz]
    
    % State-Space Matrix (positions and orientations only)
    A = [
        1, 0, 0, 0, 0, 0; % Px
        0, 1, 0, 0, 0, 0; % Py
        0, 0, 1, 0, 0, 0; % Pz
        0, 0, 0, 1, 0, 0; % α
        0, 0, 0, 0, 1, 0; % β
        0, 0, 0, 0, 0, 1; % γ
    ];
    
    % Input Matrix (positions and orientations only)
    B = [
        dT^2 / (2 * m), 0, 0, 0, 0, 0; % Px
        0, dT^2 / (2 * m), 0, 0, 0, 0; % Py
        0, 0, dT^2 / (2 * m), 0, 0, 0; % Pz
        0, 0, 0, dT^2 / (2 * Ixx), 0, 0; % α
        0, 0, 0, 0, dT^2 / (2 * Iyy), 0; % β
        0, 0, 0, 0, 0, dT^2 / (2 * Izz); % γ
    ];
    
    % Output Matrix (positions and orientations only)
    C = eye(6); % Direct mapping of states to outputs

    D = zeros(6, 6); % No direct feedthrough
    
    % State-Space equations
    xdot = A * x + B * u; % State derivative
    y = C * x + D *u;           % Output
end

== matlab function GammaandTorqueMover/Disturbance added/Linear MPC plus D/MLPM Plant1/PINV/GAMMA ==
  data: input input; position input; output output; TAU input; BETA_K input; ALPHA_X input; ALPHA_Y input; ALPHA_Z input; ALPHA_M1 input; ALPHA_M2 input; BETA_M1 input; BETA_M2 input; ALPHA_RZ input; PI input
function output = computeGammaPinvBlock(input,position,TAU,BETA_K,ALPHA_X,ALPHA_Y,ALPHA_Z,ALPHA_M1,ALPHA_M2,BETA_M1,BETA_M2,ALPHA_RZ,PI)
    % Call the generated function to compute Gamma
    X_M = position(1);
    Y_M = position(2);
    Z_M = position(3);
    ALPHA_ROTATION_M = position(4);
    BETA_ROTATION_M = position(5);
    GAMMA_ROTATION_M = position(6);
    Gamma = computeFullGammawithTorqueR4(X_M,Y_M,Z_M,ALPHA_ROTATION_M,BETA_ROTATION_M,GAMMA_ROTATION_M,TAU,BETA_K,ALPHA_X,ALPHA_Y,ALPHA_Z,ALPHA_M1,ALPHA_M2,BETA_M1,BETA_M2,ALPHA_RZ,PI);
    Gamma_pinv = pinv(Gamma);
    
    % Multiply Gamma by the input
    output =Gamma_pinv * input ;
end

== matlab function GammaandTorqueMover/Disturbance added/Linear MPC plus D/Subsystem/Gamma/GAMMA ==
  data: input input; position input; output output; TAU input; BETA_K input; ALPHA_X input; ALPHA_Y input; ALPHA_Z input; ALPHA_M1 input; ALPHA_M2 input; BETA_M1 input; BETA_M2 input; ALPHA_RZ input; PI input
function output = computeGammaBlock(input, position,TAU,BETA_K,ALPHA_X,ALPHA_Y,ALPHA_Z,ALPHA_M1,ALPHA_M2,BETA_M1,BETA_M2,ALPHA_RZ,PI)
% Call the generated function to compute Gamma
    X_M = position(1);
    Y_M = position(2);
    Z_M = position(3);
    ALPHA_ROTATION_M = position(4);
    BETA_ROTATION_M = position(5);
    GAMMA_ROTATION_M = position(6);
    Gamma = computeFullGammawithTorqueR4(X_M,Y_M,Z_M,ALPHA_ROTATION_M,BETA_ROTATION_M,GAMMA_ROTATION_M,TAU,BETA_K,ALPHA_X,ALPHA_Y,ALPHA_Z,ALPHA_M1,ALPHA_M2,BETA_M1,BETA_M2,ALPHA_RZ,PI);

    % Multiply Gamma by the input
    output = Gamma *input;
end

== matlab function GammaandTorqueMover/Disturbance added/Linear MPC plus D/Subsystem/MATLAB Function ==
  data: xdot output; u input; y output; x input
function [xdot, y] = System_SS_Model(u, x)
    % Parameters
    m = 6.6;            % Mass (kg)
    g = 9.81;           % Gravitational acceleration (m/s^2)
    
    % Moment of Inertia
    Ixx = 0.059;        % Moment of inertia around x-axis
    Iyy = 0.059;        % Moment of inertia around y-axis
    Izz = 0.12;         % Moment of inertia around z-axis
    
    % State vector x = [Px, Vx, Py, Vy, Pz, Vz, α, ω_x, β, ω_y, γ, ω_z]
    % Input vector u = [Fx, Fy, Fz, Tx, Ty, Tz]
    
    % State-Space Matrix (continuous time)
    A = zeros(12, 12);
    % Position-velocity couplings
    A(1,2) = 1;  % Px dot = Vx
    A(3,4) = 1;  % Py dot = Vy
    A(5,6) = 1;  % Pz dot = Vz
    A(7,8) = 1;  % α dot = ω_x
    A(9,10) = 1; % β dot = ω_y
    A(11,12) = 1;% γ dot = ω_z
    
    % Input Matrix (continuous time)
    B = zeros(12, 6);
    % Force to acceleration conversion
    B(2,1) = 1/m;    % Fx -> ax
    B(4,2) = 1/m;    % Fy -> ay
    B(6,3) = 1/m;    % Fz -> az
    % Torque to angular acceleration conversion
    B(8,4) = 1/Ixx;  % Tx -> α_ddot
    B(10,5) = 1/Iyy; % Ty -> β_ddot
    B(12,6) = 1/Izz; % Tz -> γ_ddot
    
    % Gravitational effect (constant acceleration in z direction)
    gravity = zeros(12,1);
    gravity(6) = -g;  % Acceleration in z direction
    
    % State derivative (continuous time)
    xdot = A * x + B * u + gravity;
    
    % Output equation: Only positions and orientations
    % Positions: Px (x(1)), Py (x(3)), Pz (x(5))
    % Orientations: α (x(7)), β (x(9)), γ (x(11))
    y = [ x(1); x(3); x(5); x(7); x(9); x(11) ];
end

== matlab function GammaandTorqueMover/Disturbance added/Linear MPC plus D/Subsystem/PINV/GAMMA ==
  data: input input; position input; output output; TAU input; BETA_K input; ALPHA_X input; ALPHA_Y input; ALPHA_Z input; ALPHA_M1 input; ALPHA_M2 input; BETA_M1 input; BETA_M2 input; ALPHA_RZ input; PI input
function output = computeGammaPinvBlock(input,position,TAU,BETA_K,ALPHA_X,ALPHA_Y,ALPHA_Z,ALPHA_M1,ALPHA_M2,BETA_M1,BETA_M2,ALPHA_RZ,PI)
    % Call the generated function to compute Gamma
    X_M = position(1);
    Y_M = position(2);
    Z_M = position(3);
    ALPHA_ROTATION_M = position(4);
    BETA_ROTATION_M = position(5);
    GAMMA_ROTATION_M = position(6);
    Gamma = computeFullGammawithTorqueR4(X_M,Y_M,Z_M,ALPHA_ROTATION_M,BETA_ROTATION_M,GAMMA_ROTATION_M,TAU,BETA_K,ALPHA_X,ALPHA_Y,ALPHA_Z,ALPHA_M1,ALPHA_M2,BETA_M1,BETA_M2,ALPHA_RZ,PI);
    Gamma_pinv = pinv(Gamma);
    
    % Multiply Gamma by the input
    output =Gamma_pinv * input ;
end

== matlab function GammaandTorqueMover/Linear MPC old/MATLAB Function ==
  data: xdot output; u input; y output; x input
function [xdot, y] = System_SS_Model(u,x)
    % Parameters
    m = 6.6;            % Mass (kg)
    dT = 0.1;           % Time step
    
    % Moment of Inertia (example values, should be calibrated to specific system)
    Ixx = 0.059;          % Moment of inertia around x-axis
    Iyy = 0.059;          % Moment of inertia around y-axis
    Izz = 0.12;         % Moment of inertia around z-axis
    
    % State vector x = [Px, Py, Pz, α, β, γ]
    % Input vector u = [Fx, Fy, Fz, Tx, Ty, Tz]
    
    % State-Space Matrix (positions and orientations only)
    A = [
        1, 0, 0, 0, 0, 0; % Px
        0, 1, 0, 0, 0, 0; % Py
        0, 0, 1, 0, 0, 0; % Pz
        0, 0, 0, 1, 0, 0; % α
        0, 0, 0, 0, 1, 0; % β
        0, 0, 0, 0, 0, 1; % γ
    ];
    
    % Input Matrix (positions and orientations only)
    B = [
        dT^2 / (2 * m), 0, 0, 0, 0, 0; % Px
        0, dT^2 / (2 * m), 0, 0, 0, 0; % Py
        0, 0, dT^2 / (2 * m), 0, 0, 0; % Pz
        0, 0, 0, dT^2 / (2 * Ixx), 0, 0; % α
        0, 0, 0, 0, dT^2 / (2 * Iyy), 0; % β
        0, 0, 0, 0, 0, dT^2 / (2 * Izz); % γ
    ];
    
    % Output Matrix (positions and orientations only)
    C = eye(6); % Direct mapping of states to outputs

    D = zeros(6, 6); % No direct feedthrough
    
    % State-Space equations
    xdot = A * x + B * u; % State derivative
    y = C * x + D *u;           % Output
end

== matlab function GammaandTorqueMover/Disturbance added/PID plus D/MLPM Plant1/Gamma/GAMMA ==
  data: input input; position input; output output; TAU input; BETA_K input; ALPHA_X input; ALPHA_Y input; ALPHA_Z input; ALPHA_M1 input; ALPHA_M2 input; BETA_M1 input; BETA_M2 input; ALPHA_RZ input; PI input
function output = computeGammaBlock(input, position,TAU,BETA_K,ALPHA_X,ALPHA_Y,ALPHA_Z,ALPHA_M1,ALPHA_M2,BETA_M1,BETA_M2,ALPHA_RZ,PI)
% Call the generated function to compute Gamma
    X_M = position(1);
    Y_M = position(2);
    Z_M = position(3);
    ALPHA_ROTATION_M = position(4);
    BETA_ROTATION_M = position(5);
    GAMMA_ROTATION_M = position(6);
    Gamma = computeFullGammawithTorqueR4(X_M,Y_M,Z_M,ALPHA_ROTATION_M,BETA_ROTATION_M,GAMMA_ROTATION_M,TAU,BETA_K,ALPHA_X,ALPHA_Y,ALPHA_Z,ALPHA_M1,ALPHA_M2,BETA_M1,BETA_M2,ALPHA_RZ,PI);

    % Multiply Gamma by the input
    output = Gamma *input;
end
